simulink model "Tfmodel"  (R2020a)
settings: Solver=VariableStepAuto  StartTime=0.0  StopTime=10.0  RelTol=1e-3
undefined symbols (not defined in the file): A_fc, Cp_f, f, mf, Po, Ufc
settings Model: Creator=marce  LastModifiedBy=tkdmc

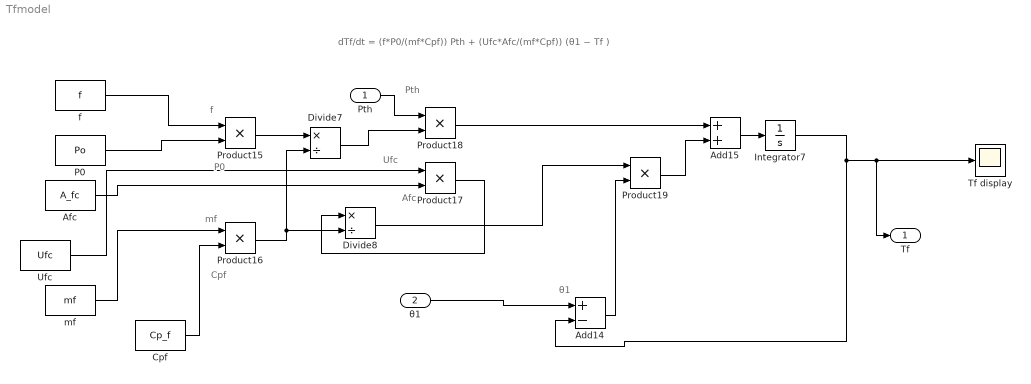
== system Tfmodel ==
  note: Ufc
  note: Afc
  note: Pth
  note: Cpf
  note: f
  note: mf
  note: P0
  note: θ1
  note: dTf/dt = (f*P0/(mf*Cpf)) Pth + (Ufc*Afc/(mf*Cpf)) (θ1 − Tf )
  Pth : Inport
  θ1 : Inport  Port=2
  Add14 : Sum  Inputs=+-
  Add15 : Sum
  Afc : Constant  Value=A_fc
  Cpf : Constant  Value=Cp_f
  Divide7 : Product  Inputs=*/
  Divide8 : Product  Inputs=*/
  Integrator7 : Integrator
  P0 : Constant  Value=Po
  Product{15..19} (5 alike) : Product
  Tf display : Scope
  Ufc : Constant  Value=Ufc
  f : Constant  Value=f
  mf : Constant  Value=mf
  Tf : Outport
  wires:
  Product15/1 -> Divide7/1
  Product17/1 -> Divide8/1
  Product16/1 -> Divide7/2, Divide8/2
  Product19/1 -> Add15/2
  Divide7/1 -> Product18/2
  Product18/1 -> Add15/1
  Integrator7/1 -> Tf/1, Tf display/1, Add14/2
  Add14/1 -> Product19/2
  Add15/1 -> Integrator7/1
  Divide8/1 -> Product19/1
  f/1 -> Product15/1
  P0/1 -> Product15/2
  Pth/1 -> Product18/1
  Afc/1 -> Product17/2
  Ufc/1 -> Product17/1
  mf/1 -> Product16/1
  Cpf/1 -> Product16/2
  θ1/1 -> Add14/1
